simulink model "EvitarObstaculo"  (R2019b)
settings: Solver=VariableStepAuto  StartTime=0.0  StopTime=10.0  RelTol=1e-3
model workspace (MAT data in the model file):
  obsx = Simulink.Parameter
  obsx.DataType = 'auto'
  obsx.Dimensions = [0 0]
  obsy = Simulink.Parameter
  obsy.DataType = 'auto'
  obsy.Dimensions = [0 0]
values from neighbouring files (symbols this model uses):
  obsx = 2.5    [part2.m]
  obsy = 2.5    [part2.m]
  refx = 10*rand-5    [part1.m]    (also in part2.m = 5)
  refy = 10*rand-5    [part1.m]    (also in part2.m = 5)
undefined symbols (not defined in the file or in its folder): DiscIntNeverNeededParam
libraries: fuzblock x1, simulink x1
settings Model: Creator=Laura  LastModifiedBy=Pablo
settings DataIOCC: ReturnWorkspaceOutputs=off

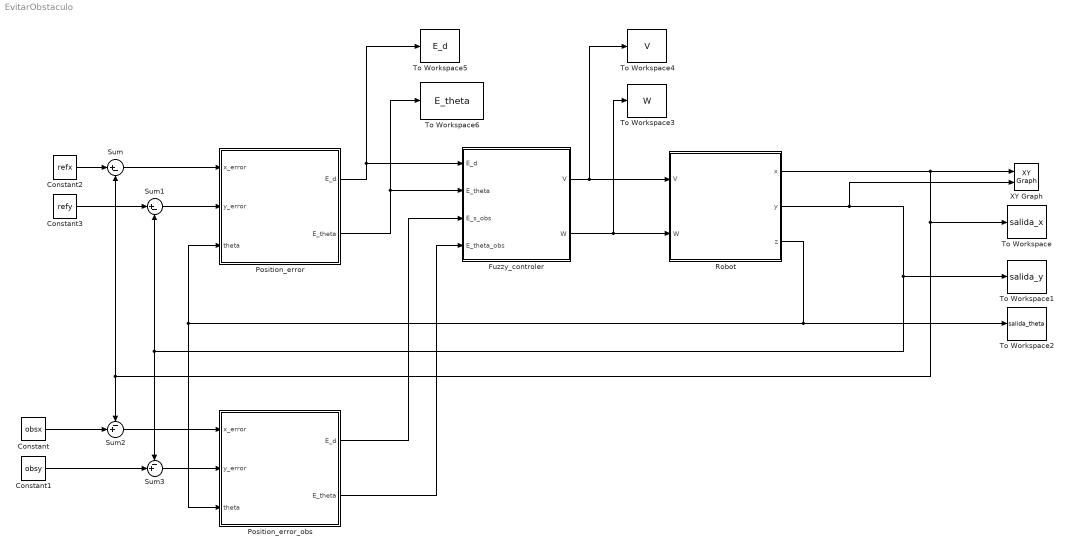
== system EvitarObstaculo ==
  Constant : Constant  Value=obsx
  Constant1 : Constant  Value=obsy
  Constant2 : Constant  Value=refx
  Constant3 : Constant  Value=refy
  Fuzzy_controler : Subsystem
  "Position_error " : Subsystem
  Position_error_obs : Subsystem
  Robot : Subsystem
  Sum : Sum  Inputs=|+-
  Sum1 : Sum  Inputs=|+-
  Sum2 : Sum  Inputs=-+|
  Sum3 : Sum  Inputs=-+|
  To Workspace : ToWorkspace  VariableName=salida_x  SaveFormat=Structure With Time  SampleTime=-1
      settings: Save2DSignal=2-D array (concatenate along first dimension)
  To Workspace1 : ToWorkspace  VariableName=salida_y  SaveFormat=Structure With Time  SampleTime=-1
      settings: Save2DSignal=2-D array (concatenate along first dimension)
  To Workspace2 : ToWorkspace  VariableName=salida_theta  SaveFormat=Structure With Time  SampleTime=-1
      settings: Save2DSignal=2-D array (concatenate along first dimension)
  To Workspace3 : ToWorkspace  VariableName=W  SaveFormat=Structure With Time  SampleTime=-1
      settings: Save2DSignal=2-D array (concatenate along first dimension)
  To Workspace4 : ToWorkspace  VariableName=V  SaveFormat=Structure With Time  SampleTime=-1
      settings: Save2DSignal=2-D array (concatenate along first dimension)
  To Workspace5 : ToWorkspace  VariableName=E_d  SaveFormat=Structure With Time  SampleTime=-1
      settings: Save2DSignal=2-D array (concatenate along first dimension)
  To Workspace6 : ToWorkspace  VariableName=E_theta  SaveFormat=Structure With Time  SampleTime=-1
      settings: Save2DSignal=2-D array (concatenate along first dimension)
  XY Graph : simulink/Sinks/XY Graph  xmin=-10  xmax=10  ymin=-10  ymax=10  st=-1
  wires:
  Sum1/1 -> "Position_error "/2("y_error ")
  Robot/3(z) -> Position_error_obs/3("theta "), "Position_error "/3("theta "), To Workspace2/1
  "Position_error "/1(E_d) -> Fuzzy_controler/1(E_d), To Workspace5/1
  Fuzzy_controler/1(V) -> Robot/1("V "), To Workspace4/1
  Fuzzy_controler/2(W) -> To Workspace3/1, Robot/2("W ")
  Robot/1(x) -> XY Graph/1, Sum2/1, Sum/2, To Workspace/1
  Sum/1 -> "Position_error "/1("x_error ")
  "Position_error "/2(E_theta) -> Fuzzy_controler/2(E_theta), To Workspace6/1
  Robot/2(y) -> XY Graph/2, Sum1/2, Sum3/1, To Workspace1/1
  Sum2/1 -> Position_error_obs/1("x_error ")
  Sum3/1 -> Position_error_obs/2("y_error ")
  Position_error_obs/1(E_d) -> Fuzzy_controler/3(E_s_obs)
  Position_error_obs/2(E_theta) -> Fuzzy_controler/4(E_theta_obs)
  Constant/1 -> Sum2/2
  Constant1/1 -> Sum3/2
  Constant2/1 -> Sum/1
  Constant3/1 -> Sum1/1

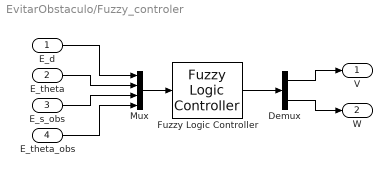
== system EvitarObstaculo/Fuzzy_controler ==
  E_d : Inport
  E_theta : Inport  Port=2
  E_s_obs : Inport  Port=3
  E_theta_obs : Inport  Port=4
  Demux : Demux  Outputs=2
  Fuzzy Logic Controller : fuzblock/Fuzzy Logic  Controller  FIS='ControlBorrosoObs.fis'  OutputSampleNumber=101  DataType=double  FuzzifiedInputs=off  RuleFiringStrengths=off  RuleOutputs=off  AggregatedOutputs=off  SimulateUsing=Interpreted execution  OutOfRangeInputValueMessage=warning  NoRuleFiredMessage=warning  EmptyOutputFuzzySetMessage=warning
  Mux : Mux
  V : Outport
  W : Outport  Port=2
  wires:
  E_d/1 -> Mux/1
  E_s_obs/1 -> Mux/3
  Demux/2 -> W/1
  E_theta_obs/1 -> Mux/4
  Mux/1 -> Fuzzy Logic Controller/1
  Demux/1 -> V/1
  Fuzzy Logic Controller/1 -> Demux/1
  E_theta/1 -> Mux/2

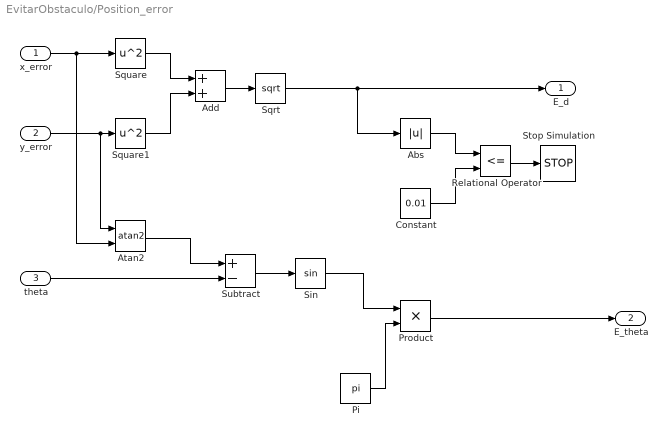
== system EvitarObstaculo/Position_error  ==
  "x_error " : Inport
  "y_error " : Inport  Port=2
  "theta " : Inport  Port=3
  Abs : Abs
  Add : Sum
  Atan2 : Trigonometry  Operator=atan2
  Constant : Constant  Value=0.01
  Pi : Constant  Value=pi  OutDataTypeStr=Inherit: Inherit via back propagation
  Product : Product
  Relational Operator : RelationalOperator  Operator=<=  OutDataTypeStr=boolean  RndMeth=Simplest
  Sin : Trigonometry
  Sqrt : Sqrt  SaturateOnIntegerOverflow=on
  Square : Math  Operator=square  SignedPower=off  SaturateOnIntegerOverflow=on
  Square1 : Math  Operator=square  SignedPower=off  SaturateOnIntegerOverflow=on
  Stop Simulation : Stop
  Subtract : Sum  Inputs=+-
  E_d : Outport
  E_theta : Outport  Port=2
  wires:
  Abs/1 -> Relational Operator/1
  Constant/1 -> Relational Operator/2
  Relational Operator/1 -> Stop Simulation/1
  "x_error "/1 -> Atan2/2, Square/1
  "y_error "/1 -> Atan2/1, Square1/1
  Square/1 -> Add/1
  Square1/1 -> Add/2
  Add/1 -> Sqrt/1
  Atan2/1 -> Subtract/1
  "theta "/1 -> Subtract/2
  Sqrt/1 -> E_d/1, Abs/1
  Subtract/1 -> Sin/1
  Sin/1 -> Product/1
  Pi/1 -> Product/2
  Product/1 -> E_theta/1

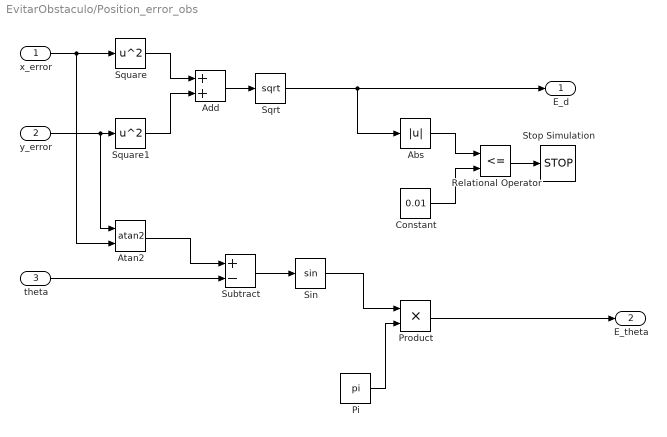
== system EvitarObstaculo/Position_error_obs ==
  "x_error " : Inport
  "y_error " : Inport  Port=2
  "theta " : Inport  Port=3
  Abs : Abs
  Add : Sum
  Atan2 : Trigonometry  Operator=atan2
  Constant : Constant  Value=0.01
  Pi : Constant  Value=pi  OutDataTypeStr=Inherit: Inherit via back propagation
  Product : Product
  Relational Operator : RelationalOperator  Operator=<=  OutDataTypeStr=boolean  RndMeth=Simplest
  Sin : Trigonometry
  Sqrt : Sqrt  SaturateOnIntegerOverflow=on
  Square : Math  Operator=square  SignedPower=off  SaturateOnIntegerOverflow=on
  Square1 : Math  Operator=square  SignedPower=off  SaturateOnIntegerOverflow=on
  Stop Simulation : Stop
  Subtract : Sum  Inputs=+-
  E_d : Outport
  E_theta : Outport  Port=2
  wires:
  Abs/1 -> Relational Operator/1
  Constant/1 -> Relational Operator/2
  Relational Operator/1 -> Stop Simulation/1
  "x_error "/1 -> Atan2/2, Square/1
  "y_error "/1 -> Atan2/1, Square1/1
  Square/1 -> Add/1
  Square1/1 -> Add/2
  Add/1 -> Sqrt/1
  Atan2/1 -> Subtract/1
  "theta "/1 -> Subtract/2
  Sqrt/1 -> E_d/1, Abs/1
  Subtract/1 -> Sin/1
  Sin/1 -> Product/1
  Pi/1 -> Product/2
  Product/1 -> E_theta/1

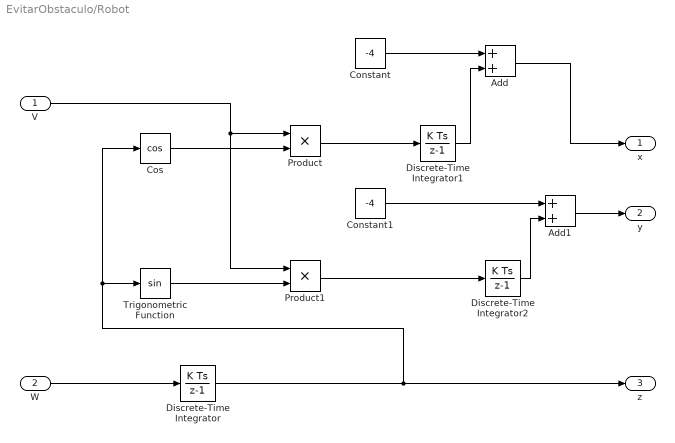
== system EvitarObstaculo/Robot ==
  "V " : Inport
  "W " : Inport  Port=2
  Add : Sum
  Add1 : Sum
  Constant : Constant  Value=-4
  Constant1 : Constant  Value=-4
  Cos : Trigonometry  Operator=cos
  Discrete-Time Integrator : DiscreteIntegrator  SampleTime=-1  ICPrevOutput=DiscIntNeverNeededParam  ICPrevScaledInput=DiscIntNeverNeededParam
  Discrete-Time Integrator1 : DiscreteIntegrator  SampleTime=-1  ICPrevOutput=DiscIntNeverNeededParam  ICPrevScaledInput=DiscIntNeverNeededParam
  Discrete-Time Integrator2 : DiscreteIntegrator  SampleTime=-1  ICPrevOutput=DiscIntNeverNeededParam  ICPrevScaledInput=DiscIntNeverNeededParam
  Product : Product
  Product1 : Product
  Trigonometric Function : Trigonometry
  x : Outport
  y : Outport  Port=2
  z : Outport  Port=3
  wires:
  Product/1 -> Discrete-Time Integrator1/1
  Trigonometric Function/1 -> Product1/2
  Discrete-Time Integrator/1 -> Cos/1, Trigonometric Function/1, z/1
  "W "/1 -> Discrete-Time Integrator/1
  Product1/1 -> Discrete-Time Integrator2/1
  Cos/1 -> Product/2
  "V "/1 -> Product1/1, Product/1
  Discrete-Time Integrator1/1 -> Add/2
  Constant/1 -> Add/1
  Add/1 -> x/1
  Constant1/1 -> Add1/1
  Discrete-Time Integrator2/1 -> Add1/2
  Add1/1 -> y/1
